simulink model "test_2dairframe"  (R2022a)
settings: Solver=VariableStepAuto  StartTime=0.0  StopTime=SimTime  RelTol=1e-3
PreLoadFcn:
  | airframe_init
values from neighbouring files (symbols this model uses):
  pose_ini = [0, 0, 0]    [airframe_init.m]
  rot_ini = [0, deg2rad(20), 0]    [airframe_init.m]
libraries: simulink x2, shared6dof x1
settings Model: Creator=amani  LastModifiedBy=amani

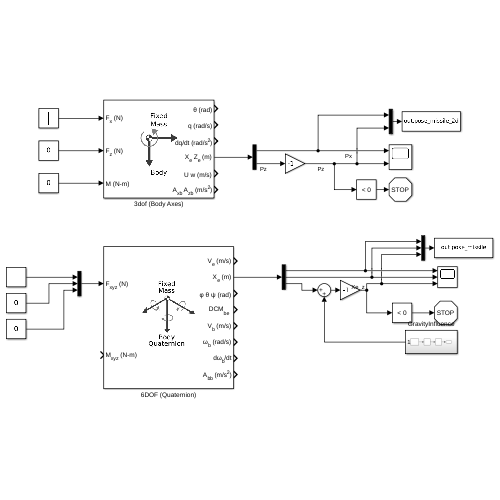
[thumbnail: Simulink's stored preview of the top-level diagram]
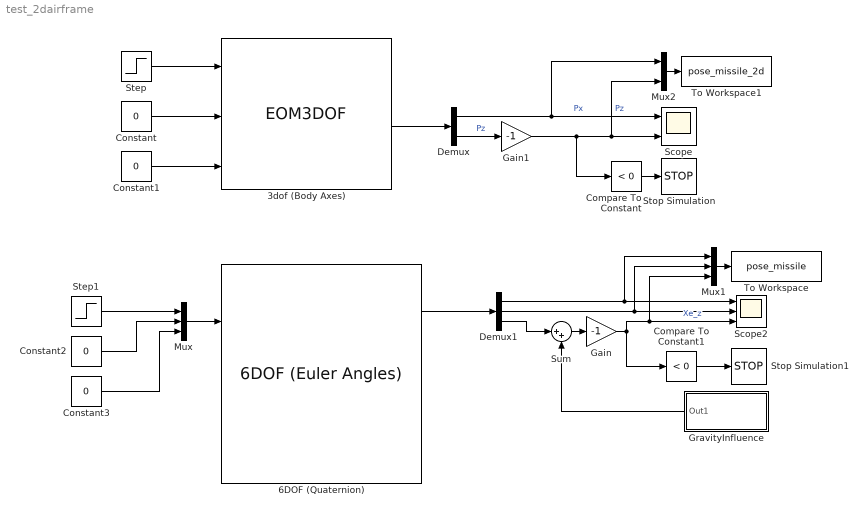
== system test_2dairframe ==
  3dof (Body Axes) : EOM3DOF  v_ini=0  theta_ini=rot_ini(2)  pos_ini=[pose_ini(1) pose_ini(3)]  mass=mass  Iyy=iyy
  6DOF (Quaternion) : shared6dof/6DOF (Euler Angles)  units=Metric (MKS)  mtype=Fixed  rep=Quaternion  xme_0=pose_ini  Vm_0=vel_ini  eul_0=rot_ini  pm_0=rotvel_ini  mass_0=mass  mass_e=0.5  mass_f=2.0  inertia=inertia  inertia_e=eye(3)  inertia_f=2*eye(3)  k_quat=1.0  vre_flag=on  abi_flag=off  aMode=0  xme_statename=''  Vm_statename=''  eul_statename=''  quat_statename=''  pm_statename=''  mass_statename=''
      settings: SourceProductBaseCode=AE,PW,DR,MT,VE
  Compare To Constant : simulink/Logic and Bit Operations/Compare To Constant  relop=<  const=0  OutDataTypeStr=boolean
  Compare To Constant1 : simulink/Logic and Bit Operations/Compare To Constant  relop=<  const=0  OutDataTypeStr=boolean
  Constant{,1..3} (4 alike) : Constant  Value=0
  Demux : Demux  Outputs=2
  Demux1 : Demux  Outputs=3
  Gain : Gain  Gain=-1
  Gain1 : Gain  Gain=-1
  GravityInfluence : Subsystem
  Mux : Mux  Inputs=3
  Mux1 : Mux  Inputs=3
  Mux2 : Mux  Inputs=2
  Scope : Scope  NumInputPorts=2
  Scope2 : Scope  NumInputPorts=3
  Step : Step  Time=2  Before=70000  After=0  SampleTime=0
  Step1 : Step  Time=2  Before=70000  After=0  SampleTime=0
  Stop Simulation : Stop
  Stop Simulation1 : Stop
  Sum : Sum  Inputs=|++
  To Workspace : ToWorkspace  VariableName=pose_missile  SaveFormat=Structure With Time  SampleTime=-1
  To Workspace1 : ToWorkspace  VariableName=pose_missile_2d  SaveFormat=Structure With Time  SampleTime=-1
  wires:
  3dof (Body Axes)/4 -> Demux/1
  Demux/1 -> Mux2/1, Scope/1  "Px"
  Constant1/1 -> 3dof (Body Axes)/3
  Compare To Constant/1 -> Stop Simulation/1
  Demux/2 -> Gain1/1  "Pz"
  Gain1/1 -> Compare To Constant/1, Mux2/2, Scope/2  "Pz"
  Constant/1 -> 3dof (Body Axes)/2
  Step/1 -> 3dof (Body Axes)/1
  Demux1/1 -> Mux1/1, Scope2/1
  Gain/1 -> Mux1/3, Scope2/3, Compare To Constant1/1  "Xe_z"
  Mux/1 -> 6DOF (Quaternion)/1
  Sum/1 -> Gain/1
  Constant2/1 -> Mux/2
  Demux1/3 -> Sum/1
  GravityInfluence/1(Out1) -> Sum/2
  Compare To Constant1/1 -> Stop Simulation1/1
  Constant3/1 -> Mux/3
  Mux1/1 -> To Workspace/1
  Step1/1 -> Mux/1
  6DOF (Quaternion)/2 -> Demux1/1
  Demux1/2 -> Mux1/2, Scope2/2
  Mux2/1 -> To Workspace1/1

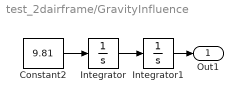
== system test_2dairframe/GravityInfluence ==
  Constant2 : Constant  Value=9.81
  Integrator : Integrator
  Integrator1 : Integrator
  Out1 : Outport
  wires:
  Integrator/1 -> Integrator1/1
  Constant2/1 -> Integrator/1
  Integrator1/1 -> Out1/1
